simulink model "fsae_bike_model"  (R2023a)
settings: Solver=VariableStepAuto  StartTime=0.0  StopTime=10.0  RelTol=1e-3
InitFcn:
  | load("data/refPath.mat")
undefined symbols (not defined in the file): angulo_inicial_graus, distancia_eixo_ftraseiro_centro_massa, massa, pos_inicial_x, pos_inicial_y, velt_res
libraries: vehdynlibviscommon x1, simulink_extras x1, autolibshared x1
settings Model: DataDictionary=fsae_bike_model23a.sldd  Creator=rodri  LastModifiedBy=thailon
settings RTWCC: GPUComputeCapability=5.0

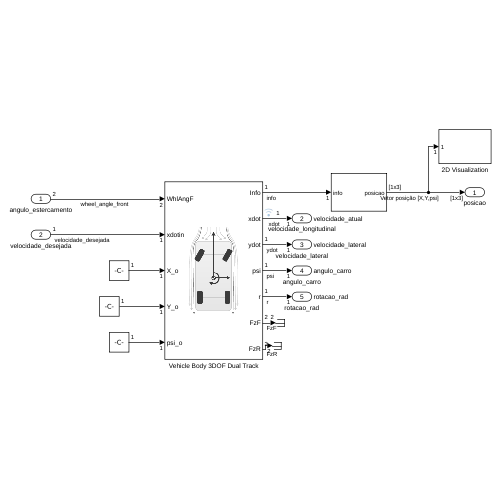
[thumbnail: Simulink's stored preview of the top-level diagram]
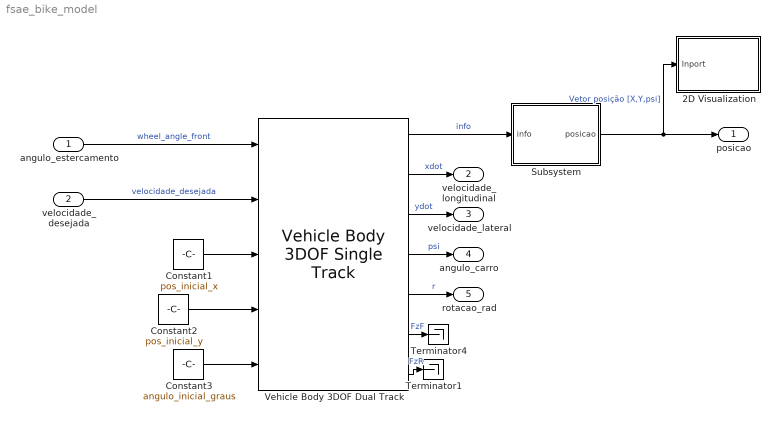
== system fsae_bike_model ==
  angulo_estercamento : Inport
  velocidade_desejada : Inport  Port=2
  2D Visualization : Subsystem
  Constant1 : Constant  Value=pos_inicial_x
  Constant2 : Constant  Value=pos_inicial_y
  Constant3 : Constant  Value=angulo_inicial_graus
  Subsystem : Subsystem
  Terminator1 : Terminator
  Terminator4 : Terminator
  Vehicle Body 3DOF Dual Track : autolibshared/Vehicle Body 3DOF Single Track  trackMode=Dual  inputMode=External longitudinal velocity  frontSteerMode=on  rearSteerMode=off  windMode=off  muMode=off  extFMode=off  extMMode=off  htchFMode=off  htchMMode=off  extXo=on  extpsio=on  extxdoto=off  extro=off  extYo=on  extTamb=off  extydoto=off  aMode=2  NF=numero_de_eixos_frente  NR=numero_de_eixos_traseira  m=massa  a=distancia_eixo_frontal_centro_massa  b=distancia_eixo_ftraseiro_centro_massa  h=distancia_chao_plano_centro_massa  dh=1  hh=0.2  X_o=0  xdot_o=velt_res(1)  CalphaMode=off  sigmaMode=on  d=distancia_lateral_linha_gemetrica_centro_massa  hl=0  w=bitola  Cy_f=rigidez_lateral_pneu_frontal  Cy_r=rigidez_lateral_pneu_traseira  sigma_f=comprimento_relaxacao_frontal  sigma_r=comprimento_relaxacao_traseira  alpha_f_brk=[-.1 .1]  Cy_f_data=[-9e3 9e3]  alpha_r_brk=[-.1 .1]  Cy_r_data=[-9e3 9e3]  Y_o=0  ydot_o=velocidade_inicial  Izz=inercial_polar_yaw  psi_o=0  r_o=giro_yaw_inicial  Af=area_arrasto_longitudinal  Cd=coeficiente_longitudinal_arrasto  Cl=coefficient_longitudinal_sustentacao  Cpm=arrasto_longitudinal_pitch  beta_w=angulo_relativo_vento_vetor  Cs=vetor_coeficiente_forca_lateral  Cym=vetor_yaw_momento_coeficiente  Pabs=101325  Tair=273  g=9.81  mu=1  xdot_tol=.01  Fznom=5000  Fxtire_sat=7e4  Fytire_sat=7e4  longOff=0  latOff=0  vertOff=0  wrapAng=off
  posicao : Outport
  velocidade_longitudinal : Outport  Port=2  SignalName=velocidade_atual
  velocidade_lateral : Outport  Port=3  SignalName=velocidade_lateral
  angulo_carro : Outport  Port=4  SignalName=angulo_carro
  rotacao_rad : Outport  Port=5  SignalName=rotacao_rad
  wires:
  angulo_estercamento/1 -> Vehicle Body 3DOF Dual Track/1  "wheel_angle_front"
  Constant3/1 -> Vehicle Body 3DOF Dual Track/5
  Constant1/1 -> Vehicle Body 3DOF Dual Track/3
  velocidade_desejada/1 -> Vehicle Body 3DOF Dual Track/2  "velocidade_desejada"
  Constant2/1 -> Vehicle Body 3DOF Dual Track/4
  Vehicle Body 3DOF Dual Track/2 -> velocidade_longitudinal/1  "xdot"
  Vehicle Body 3DOF Dual Track/3 -> velocidade_lateral/1  "ydot"
  Vehicle Body 3DOF Dual Track/4 -> angulo_carro/1  "psi"
  Vehicle Body 3DOF Dual Track/5 -> rotacao_rad/1  "r"
  Subsystem/1(posicao) -> 2D Visualization/1(Inport), posicao/1  "Vetor posição [X,Y,psi]"
  Vehicle Body 3DOF Dual Track/1 -> Subsystem/1(info)  "info"
  Vehicle Body 3DOF Dual Track/6 -> Terminator4/1  "FzF"
  Vehicle Body 3DOF Dual Track/7 -> Terminator1/1  "FzR"

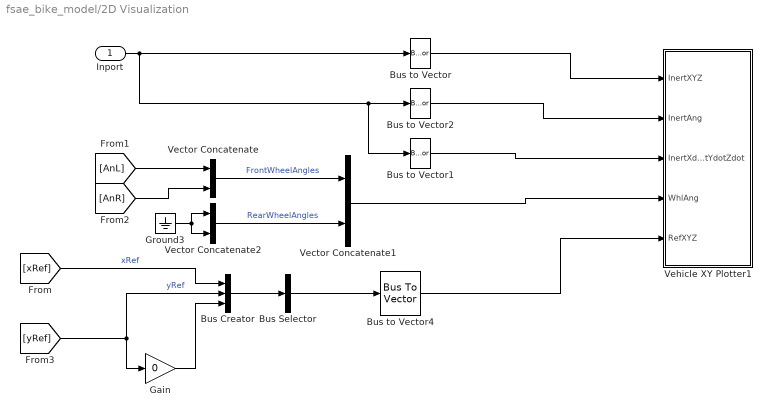
== system fsae_bike_model/2D Visualization ==
  Inport : Inport
  Bus Creator : BusCreator  Inputs=3
  Bus Selector : BusSelector  OutputSignals=xRef,yRef,signal3  OutputAsBus=on
  Bus to Vector{,1..2,4} (4 alike) : BusToVector
  Gain : Gain  Gain=0
  Ground3 : Ground
  Vector Concatenate : Concatenate
  Vector Concatenate1 : Concatenate
  Vector Concatenate2 : Concatenate
  Vehicle XY Plotter1 : Subsystem  mask(Vehicle XY Plotter){extRef=on, extStats=off, extTireF=off, a=2, b=2, w=2, figBorder=10, bufferSize=1024, velNorm=5, tireFNorm=1000, pltDT=0.2}
      mask prompts: extRef "Plot path reference, extRef"; extStats "Display speed, RPM and Gear"; extTireF "Display tire forces"; a "Distance to front axle from CG, a [m]:"; b "Distance to rear axle from CG, b [m]:"; w "Track width, w [m]:"; figBorder "Distance to figure borders, figBorder [m]:"; bufferSize "Path buffer sampe size, bufferSize []:"; velNorm "Velocity vector scaling, velNorm [m*s/m]:"; tireFNorm "Tire force vector scaling, tireFNorm [m/N]:"; pltDT "Plot update rate, pltDT [s]:"
      mask help:
      | This block will display a MATLAB figure which indicates the vehicle path, current position and heading velocity.
      | An optional path reference is also provided.
      mask init:
      | block = gcb;
      | if autoblkschecksimstopped(block)
      |     ParamNames = {'extRef';'extStats';'extTireF';'extTireF'};
      |     PortNames = {'RefXYZ';'Stats';'TireFx';'TireFy'};
      |     for idx=1:length(PortNames)
      |         InportOption  = {'built-in/Ground', [PortNames{idx}, ' Ground'];...
      |             'built-in/Inport',PortNames{idx}};
      |         if ~strcmp(get_param(block,ParamNames{idx}),'on')
      |             NewBlkHdl = autoblksreplaceblock(block, InportOption, 1);
      |             set_param(NewBlkHdl, 'ShowName', 'off');
      |         else
      |             autoblksreplaceblock(block, InportOption, 2);
      |         end
      |     end
      |     InportNames = {'InertXYZ';'InertAng';'InertXdotYdotZdot';'WhlAng';'RefXYZ';'Stats';'TireFx';'TireFy'};
      |     FoundNames = get_param(find_system(block, 'LookUnderMasks', 'all', 'SearchDepth', 1, 'FollowLinks', 'on', 'BlockType', 'Inport'), 'Name');
      |     [~,PortI] = intersect(InportNames, FoundNames);
      |     PortI = sort(PortI);
      |     for idx = 1:length(PortI)
      |         set_param([block, '/', InportNames{PortI(idx)}], 'Port', num2str(idx));
      |     end
      | end
      mask TypeOptions a: Vehicle XY Plotter/a
      mask TypeOptions b: Vehicle XY Plotter/b
      mask TypeOptions w: Vehicle XY Plotter/w
      mask TypeOptions figBorder: Vehicle XY Plotter/figBorder
      mask TypeOptions bufferSize: Vehicle XY Plotter/bufferSize
      mask TypeOptions velNorm: Vehicle XY Plotter/velNorm
      mask TypeOptions tireFNorm: Vehicle XY Plotter/tireFNorm
      mask DialogControl Container3 Prompt: Plot and Display Options
  wires:
  Bus Creator/1 -> Bus Selector/1
  [xRef] -> Bus Creator/1  "xRef"
  Gain/1 -> Bus Creator/3
  [yRef] -> Gain/1, Bus Creator/2  "yRef"
  Bus Selector/1 -> Bus to Vector4/1
  Bus to Vector4/1 -> Vehicle XY Plotter1/5(RefXYZ)
  [AnR] -> Vector Concatenate/2
  Inport/1 -> Bus to Vector/1, Bus to Vector1/1, Bus to Vector2/1
  Bus to Vector2/1 -> Vehicle XY Plotter1/2(InertAng)
  Bus to Vector/1 -> Vehicle XY Plotter1/1(InertXYZ)
  Bus to Vector1/1 -> Vehicle XY Plotter1/3(InertXdotYdotZdot)
  Vector Concatenate2/1 -> Vector Concatenate1/2  "RearWheelAngles"
  [AnL] -> Vector Concatenate/1
  Vector Concatenate/1 -> Vector Concatenate1/1  "FrontWheelAngles"
  Ground3/1 -> Vector Concatenate2/2, Vector Concatenate2/1
  Vector Concatenate1/1 -> Vehicle XY Plotter1/4(WhlAng)

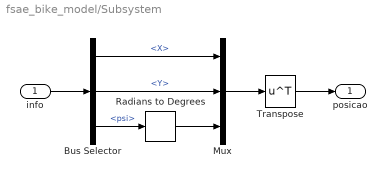
== system fsae_bike_model/Subsystem ==
  info : Inport
  Bus Selector : BusSelector  OutputSignals=InertFrm.Cg.Disp.X,InertFrm.Cg.Disp.Y,InertFrm.Cg.Ang.psi
  Mux : Mux  Inputs=3
  Radians to Degrees : simulink_extras/Transformations/Radians to Degrees
  Transpose : Math  Operator=transpose  SignedPower=on
  posicao : Outport
  wires:
  Mux/1 -> Transpose/1
  info/1 -> Bus Selector/1
  Bus Selector/1 -> Mux/1  "<X>"
  Radians to Degrees/1 -> Mux/3
  Bus Selector/2 -> Mux/2  "<Y>"
  Transpose/1 -> posicao/1
  Bus Selector/3 -> Radians to Degrees/1  "<psi>"

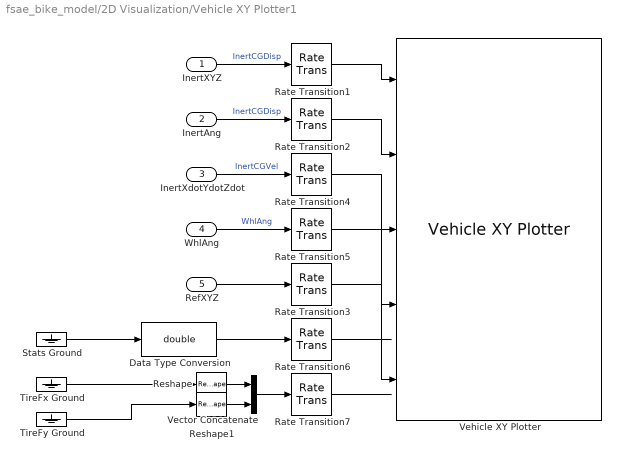
== system fsae_bike_model/2D Visualization/Vehicle XY Plotter1 ==
  InertXYZ : Inport
  InertAng : Inport  Port=2
  InertXdotYdotZdot : Inport  Port=3
  WhlAng : Inport  Port=4
  RefXYZ : Inport  Port=5
  Data Type Conversion : DataTypeConversion  OutDataTypeStr=double  SaturateOnIntegerOverflow=off  RndMeth=Floor
  Rate Transition{1..7} (7 alike) : RateTransition  Deterministic=off  OutPortSampleTime=pltDT
  Reshape : Reshape  OutputDimensionality=Row vector (2-D)
  Reshape1 : Reshape  OutputDimensionality=Row vector (2-D)
  Stats Ground : Ground
  TireFx Ground : Ground
  TireFy Ground : Ground
  Vector Concatenate : Concatenate  Mode=Multidimensional array
  Vehicle XY Plotter : vehdynlibviscommon/Vehicle XY Plotter  w=w  a=a  b=b  figBorder=figBorder  bufferSize=bufferSize  extStats=off  extTireF=off
  wires:
  TireFy Ground/1 -> Reshape1/1
  TireFx Ground/1 -> Reshape/1
  Stats Ground/1 -> Data Type Conversion/1
  InertAng/1 -> Rate Transition2/1  "InertCGDisp"
  InertXdotYdotZdot/1 -> Rate Transition4/1  "InertCGVel"
  InertXYZ/1 -> Rate Transition1/1  "InertCGDisp"
  WhlAng/1 -> Rate Transition5/1  "WhlAng"
  Rate Transition3/1 -> Vehicle XY Plotter/5
  Rate Transition1/1 -> Vehicle XY Plotter/1
  Rate Transition2/1 -> Vehicle XY Plotter/2
  Rate Transition4/1 -> Vehicle XY Plotter/3
  Rate Transition5/1 -> Vehicle XY Plotter/4
  Rate Transition6/1 -> ?
  Data Type Conversion/1 -> Rate Transition6/1
  Rate Transition7/1 -> ?
  RefXYZ/1 -> Rate Transition3/1
  Reshape/1 -> Vector Concatenate/1
  Reshape1/1 -> Vector Concatenate/2
  Vector Concatenate/1 -> Rate Transition7/1
